simulink library "robot2"
libraries: AtomicLibrary x3, BusImpl x1

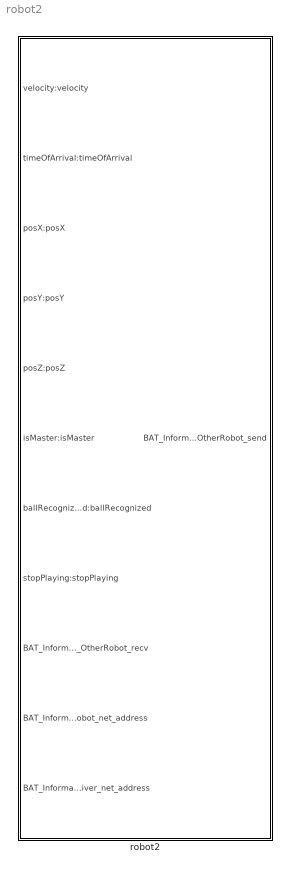
== system robot2 ==
  robot2 : Subsystem  Tag=id=_Fl7EwN8LEeKgPPszxxPBOg

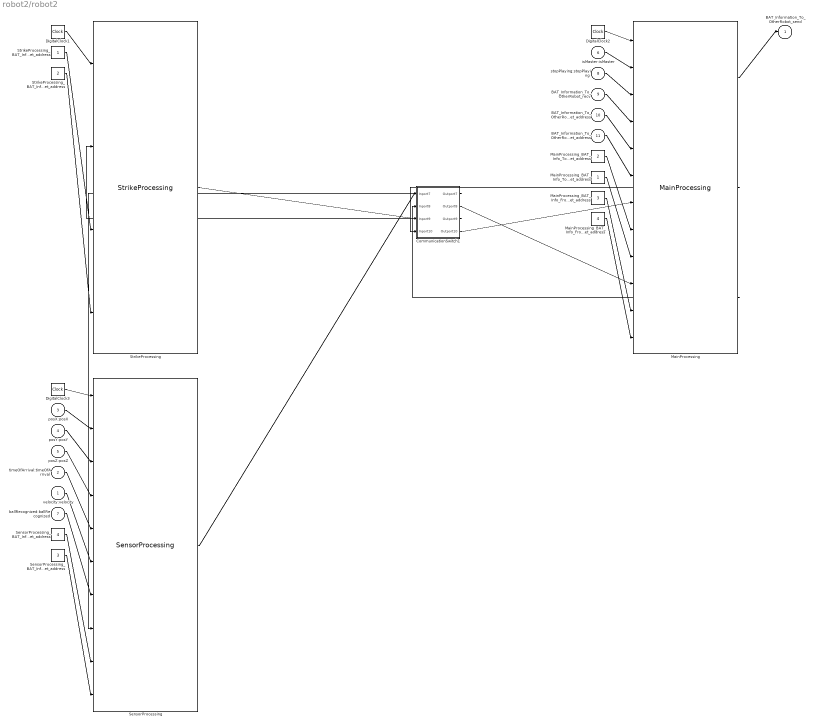
== system robot2/robot2 ==
  velocity:velocity : Inport  Tag=id=_F7pdIN8LEeKgPPszxxPBOg  Port=1  DataType=double  OutDataType=fixdt(1, 16)  OutScaling=2^0  OutDataTypeStr=double
  timeOfArrival:timeOfArrival : Inport  Tag=id=_F7z1MN8LEeKgPPszxxPBOg  Port=2  DataType=double  OutDataType=fixdt(1, 16)  OutScaling=2^0  OutDataTypeStr=double
  posX:posX : Inport  Tag=id=_F8ACcN8LEeKgPPszxxPBOg  Port=3  DataType=double  OutDataType=fixdt(1, 16)  OutScaling=2^0  OutDataTypeStr=double
  posY:posY : Inport  Tag=id=_F8OE4N8LEeKgPPszxxPBOg  Port=4  DataType=double  OutDataType=fixdt(1, 16)  OutScaling=2^0  OutDataTypeStr=double
  posZ:posZ : Inport  Tag=id=_F8ejkN8LEeKgPPszxxPBOg  Port=5  DataType=double  OutDataType=fixdt(1, 16)  OutScaling=2^0  OutDataTypeStr=double
  isMaster:isMaster : Inport  Tag=id=_F8tNEN8LEeKgPPszxxPBOg  Port=6  DataType=boolean  OutDataType=fixdt(1, 16)  OutScaling=2^0  OutDataTypeStr=boolean
  ballRecognized:ballRecognized : Inport  Tag=id=_F86ocN8LEeKgPPszxxPBOg  Port=7  DataType=boolean  OutDataType=fixdt(1, 16)  OutScaling=2^0  OutDataTypeStr=boolean
  stopPlaying:stopPlaying : Inport  Tag=id=_F9GOoN8LEeKgPPszxxPBOg  Port=8  DataType=boolean  OutDataType=fixdt(1, 16)  OutScaling=2^0  OutDataTypeStr=boolean
  BAT_Information_To_OtherRobot_recv : Inport  Tag=id=_F9i6kN8LEeKgPPszxxPBOg  Port=9  DataType=auto  OutDataType=fixdt(1, 16)  OutScaling=2^0  UseBusObject=on  OutDataTypeStr=Inherit: auto
      settings: BusObject=PacketBus
  BAT_Information_To_OtherRobot_net_address : Inport  Tag=id=_F9i6kt8LEeKgPPszxxPBOg  Port=10  DataType=uint8  OutDataType=fixdt(1, 16)  OutScaling=2^0  OutDataTypeStr=uint8
  BAT_Information_To_OtherRobot_receiver_net_address : Inport  Tag=id=_F9jhoN8LEeKgPPszxxPBOg  Port=11  DataType=uint8  OutDataType=fixdt(1, 16)  OutScaling=2^0  OutDataTypeStr=uint8
  BAT_Information_To_OtherRobot_send : Outport  Tag=id=_F9i6kd8LEeKgPPszxxPBOg  Port=1  DataType=auto  OutDataType=fixdt(1, 16)  OutScaling=2^0  UseBusObject=on  OutDataTypeStr=Inherit: auto
      settings: BusObject=PacketBus
  CommunicationSwitch1 : Subsystem  Tag=id=_Fl7Ewd8LEeKgPPszxxPBOg  LoadFcn=MainBusGenerator
  StrikeProcessing : AtomicLibrary/StrikeProcessing  Tag=id=_FmcpMN8LEeKgPPszxxPBOg
  DigitalClock1 : DigitalClock  Tag=id=_FmdQQd8LEeKgPPszxxPBOg  SampleTime=0.001
  MainProcessing : AtomicLibrary/MainProcessing  Tag=id=_FmfFcN8LEeKgPPszxxPBOg
  DigitalClock2 : DigitalClock  Tag=id=_FmfFct8LEeKgPPszxxPBOg  SampleTime=0.001
  SensorProcessing : AtomicLibrary/SensorProcessing  Tag=id=_Fmg6oN8LEeKgPPszxxPBOg
  DigitalClock3 : DigitalClock  Tag=id=_Fmhhsd8LEeKgPPszxxPBOg  SampleTime=0.001
  StrikeProcessing_BAT_Info1_net_address : Constant  Tag=id=_F44dAd8LEeKgPPszxxPBOg  Value=1  OutDataTypeMode=uint8  OutDataTypeStr=uint8
  MainProcessing_BAT_Info_ToStrikeProcessing1_net_address : Constant  Tag=id=_F5C1Ed8LEeKgPPszxxPBOg  Value=2  OutDataTypeMode=uint8  OutDataTypeStr=uint8
  MainProcessing_BAT_Info_From_SensorProcessing1_net_address : Constant  Tag=id=_F5WXEd8LEeKgPPszxxPBOg  Value=3  OutDataTypeMode=uint8  OutDataTypeStr=uint8
  SensorProcessing_BAT_Info1_net_address : Constant  Tag=id=_F5lAkd8LEeKgPPszxxPBOg  Value=4  OutDataTypeMode=uint8  OutDataTypeStr=uint8
  SensorProcessing_BAT_Info1_receiver_net_address : Constant  Tag=id=_HB9k898LEeKgPPszxxPBOg  Value=3  OutDataTypeMode=uint8  OutDataTypeStr=uint8
  MainProcessing_BAT_Info_From_SensorProcessing1_receiver_net_address : Constant  Tag=id=_HCABMd8LEeKgPPszxxPBOg  Value=4  OutDataTypeMode=uint8  OutDataTypeStr=uint8
  StrikeProcessing_BAT_Info1_receiver_net_address : Constant  Tag=id=_HCJLIN8LEeKgPPszxxPBOg  Value=2  OutDataTypeMode=uint8  OutDataTypeStr=uint8
  MainProcessing_BAT_Info_ToStrikeProcessing1_receiver_net_address : Constant  Tag=id=_HCKZQd8LEeKgPPszxxPBOg  Value=1  OutDataTypeMode=uint8  OutDataTypeStr=uint8
  wires:
  DigitalClock1/1 -> StrikeProcessing/1
  DigitalClock2/1 -> MainProcessing/1
  DigitalClock3/1 -> SensorProcessing/1
  StrikeProcessing_BAT_Info1_net_address/1 -> StrikeProcessing/3
  MainProcessing_BAT_Info_ToStrikeProcessing1_net_address/1 -> MainProcessing/8
  MainProcessing_BAT_Info_From_SensorProcessing1_net_address/1 -> MainProcessing/11
  SensorProcessing_BAT_Info1_net_address/1 -> SensorProcessing/9
  SensorProcessing/1 -> CommunicationSwitch1/1(Inport7)
  MainProcessing/3 -> CommunicationSwitch1/2(Inport8)
  CommunicationSwitch1/2(Outport8) -> MainProcessing/10
  CommunicationSwitch1/1(Outport7) -> SensorProcessing/8
  SensorProcessing_BAT_Info1_receiver_net_address/1 -> SensorProcessing/10
  MainProcessing_BAT_Info_From_SensorProcessing1_receiver_net_address/1 -> MainProcessing/12
  StrikeProcessing/1 -> CommunicationSwitch1/3(Inport9)
  MainProcessing/2 -> CommunicationSwitch1/4(Inport10)
  CommunicationSwitch1/4(Outport10) -> MainProcessing/7
  CommunicationSwitch1/3(Outport9) -> StrikeProcessing/2
  StrikeProcessing_BAT_Info1_receiver_net_address/1 -> StrikeProcessing/4
  MainProcessing_BAT_Info_ToStrikeProcessing1_receiver_net_address/1 -> MainProcessing/9
  isMaster:isMaster/1 -> MainProcessing/2
  stopPlaying:stopPlaying/1 -> MainProcessing/3
  ballRecognized:ballRecognized/1 -> SensorProcessing/7
  velocity:velocity/1 -> SensorProcessing/6
  posY:posY/1 -> SensorProcessing/3
  timeOfArrival:timeOfArrival/1 -> SensorProcessing/5
  posX:posX/1 -> SensorProcessing/2
  posZ:posZ/1 -> SensorProcessing/4
  BAT_Information_To_OtherRobot_recv/1 -> MainProcessing/4
  MainProcessing/1 -> BAT_Information_To_OtherRobot_send/1
  BAT_Information_To_OtherRobot_receiver_net_address/1 -> MainProcessing/6
  BAT_Information_To_OtherRobot_net_address/1 -> MainProcessing/5

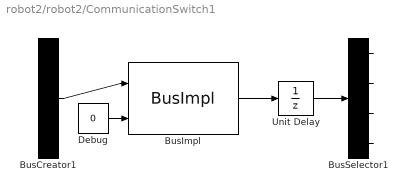
== system robot2/robot2/CommunicationSwitch1 ==
  Inport7 : Inport  Tag=id=_HB895N8LEeKgPPszxxPBOg  Port=1  DataType=auto  OutDataType=fixdt(1, 16)  OutScaling=2^0  UseBusObject=on  OutDataTypeStr=Inherit: auto
      settings: BusObject=PacketBus
  Inport8 : Inport  Tag=id=_HB9k8d8LEeKgPPszxxPBOg  Port=2  DataType=auto  OutDataType=fixdt(1, 16)  OutScaling=2^0  UseBusObject=on  OutDataTypeStr=Inherit: auto
      settings: BusObject=PacketBus
  Inport9 : Inport  Tag=id=_HCIkEt8LEeKgPPszxxPBOg  Port=3  DataType=auto  OutDataType=fixdt(1, 16)  OutScaling=2^0  UseBusObject=on  OutDataTypeStr=Inherit: auto
      settings: BusObject=PacketBus
  Inport10 : Inport  Tag=id=_HCIkFN8LEeKgPPszxxPBOg  Port=4  DataType=auto  OutDataType=fixdt(1, 16)  OutScaling=2^0  UseBusObject=on  OutDataTypeStr=Inherit: auto
      settings: BusObject=PacketBus
  Outport7 : Outport  Tag=id=_HB9k8N8LEeKgPPszxxPBOg  Port=1  DataType=auto  OutDataType=fixdt(1, 16)  OutScaling=2^0  UseBusObject=on  OutDataTypeStr=Inherit: auto
      settings: BusObject=PacketBus
  Outport8 : Outport  Tag=id=_HB9k8t8LEeKgPPszxxPBOg  Port=2  DataType=auto  OutDataType=fixdt(1, 16)  OutScaling=2^0  UseBusObject=on  OutDataTypeStr=Inherit: auto
      settings: BusObject=PacketBus
  Outport9 : Outport  Tag=id=_HCIkE98LEeKgPPszxxPBOg  Port=3  DataType=auto  OutDataType=fixdt(1, 16)  OutScaling=2^0  UseBusObject=on  OutDataTypeStr=Inherit: auto
      settings: BusObject=PacketBus
  Outport10 : Outport  Tag=id=_HCIkFd8LEeKgPPszxxPBOg  Port=4  DataType=auto  OutDataType=fixdt(1, 16)  OutScaling=2^0  UseBusObject=on  OutDataTypeStr=Inherit: auto
      settings: BusObject=PacketBus
  BusCreator1 : BusCreator  Inputs=4  UseBusObject=on
      settings: BusObject=MainBus
  BusSelector1 : BusSelector  OutputSignals=rc1,rc2,rc3,rc4
  Unit Delay : UnitDelay  SampleTime=-1
  BusImpl : BusImpl/BusImpl
  Debug : Constant  Value=0  OutDataType=fixdt(1, 16)  OutScaling=2^0
  wires:
  BusImpl/1 -> Unit Delay/1
  BusCreator1/1 -> BusImpl/1
  Unit Delay/1 -> BusSelector1/1
  Inport7/1 -> BusCreator1/1  "rc1"
  Inport8/1 -> BusCreator1/2  "rc2"
  Inport9/1 -> BusCreator1/3  "rc3"
  Inport10/1 -> BusCreator1/4  "rc4"
  BusSelector1/1 -> Outport7/1
  BusSelector1/2 -> Outport8/1
  BusSelector1/3 -> Outport9/1
  BusSelector1/4 -> Outport10/1
  Debug/1 -> BusImpl/2
